simulink model "gs_vector_test"  (R2016b)
settings: Solver=VariableStepAuto  StartTime=0.0  StopTime=19000  RelTol=1e-3
values from neighbouring files (symbols this model uses):
  fsw_params = init_fsw_params()    [gs_vector_test_init.m]
libraries: GPS_time_lib x1, ground_visualization x1, gs_prediction_lib x1, sgp4_lib_fsw x1, time_coord_rotation_lib x1
settings Model: Creator=Taylor  LastModifiedBy=evich

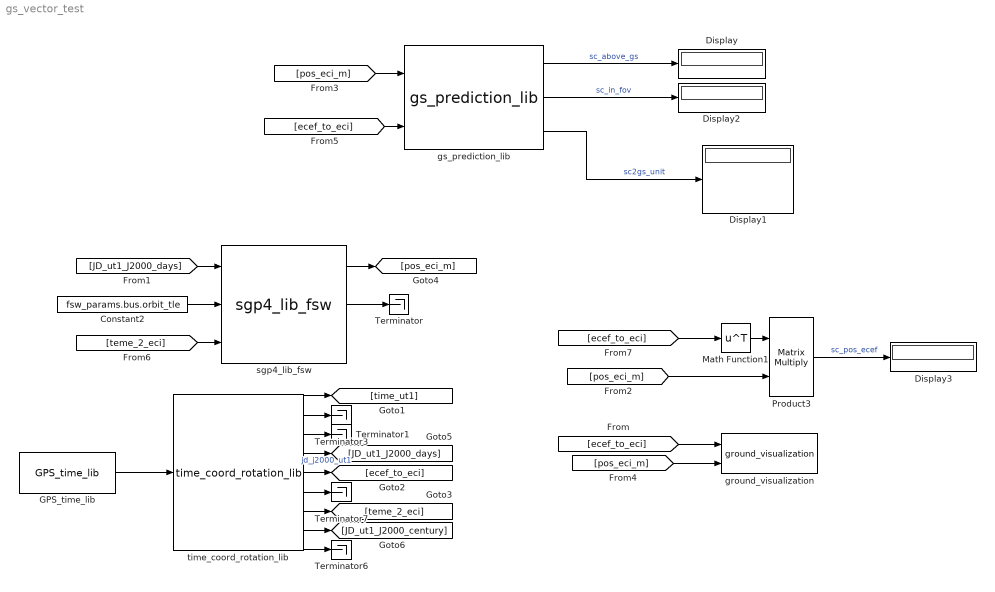
== system gs_vector_test ==
  Constant2 : Constant  Value=fsw_params.bus.orbit_tle
  Display{,1..3} (4 alike) : Display
  GPS_time_lib : GPS_time_lib/GPS_time_lib
  Math Function1 : Math  Operator=transpose  SaturateOnIntegerOverflow=on
  Product3 : Product  Multiplication=Matrix(*)
  Terminator{,1,3,6..7} (5 alike) : Terminator
  ground_visualization : ground_visualization/ground_visualization
  gs_prediction_lib : gs_prediction_lib/gs_prediction_lib
  sgp4_lib_fsw : sgp4_lib_fsw/sgp4_lib_fsw
  time_coord_rotation_lib : time_coord_rotation_lib/time_coord_rotation_lib
  wires:
  gs_prediction_lib/1 -> Display/1  "sc_above_gs"
  gs_prediction_lib/3 -> Display1/1  "sc2gs_unit"
  gs_prediction_lib/2 -> Display2/1  "sc_in_fov"
  time_coord_rotation_lib/2 -> Terminator3/1
  time_coord_rotation_lib/1 -> [time_ut1]
  [ecef_to_eci] -> ground_visualization/1
  sgp4_lib_fsw/1 -> [pos_eci_m]
  [JD_ut1_J2000_days] -> sgp4_lib_fsw/1
  sgp4_lib_fsw/2 -> Terminator/1
  GPS_time_lib/1 -> time_coord_rotation_lib/1
  [pos_eci_m] -> ground_visualization/2
  Constant2/1 -> sgp4_lib_fsw/2
  [ecef_to_eci] -> gs_prediction_lib/2
  [pos_eci_m] -> gs_prediction_lib/1
  time_coord_rotation_lib/4 -> [JD_ut1_J2000_days]  "jd_j2000_ut1"
  time_coord_rotation_lib/5 -> [ecef_to_eci]
  time_coord_rotation_lib/6 -> Terminator7/1
  time_coord_rotation_lib/7 -> [teme_2_eci]
  time_coord_rotation_lib/8 -> [JD_ut1_J2000_century]
  time_coord_rotation_lib/9 -> Terminator6/1
  time_coord_rotation_lib/3 -> Terminator1/1
  [teme_2_eci] -> sgp4_lib_fsw/3
  [ecef_to_eci] -> Math Function1/1
  Math Function1/1 -> Product3/1
  [pos_eci_m] -> Product3/2
  Product3/1 -> Display3/1  "sc_pos_ecef"
